simulink model "Demo5"  (Simulink 6.5)
settings: Solver=ode23t  SolverMode=SingleTasking  StartTime=0.0  StopTime=0.2  MaxStep=5e-5  RelTol=1e-3  AbsTol=1e-2
undefined symbols (not defined in the file): powergui
libraries: powerlib x5, powerlib_extras x2
settings Model: Creator=sybille  LastModifiedBy=PC_0  ExtModeTrigMode=oneshot  ExtModeArmWhenConnect=off  ExtModeAutoUpdateStatusClock=off  ProdHWDeviceType=Specified
settings DataIOCC: Decimation=10  LimitDataPoints=off  SaveFinalState=on  SaveOutput=off  SignalLoggingName=sigsOut
settings OptimizationCC: BlockReduction=off  BooleanDataType=off  InlineInvariantSignals=on
settings DebuggingCC: CheckExecutionContextPreStartOutputMsg=on  CheckExecutionContextRuntimeOutputMsg=on  SolverPrmCheckMsg=none  MultiTaskDSMMsg=warning  MultiTaskCondExecSysMsg=none  SigSpecEnsureSampleTimeMsg=none  UnconnectedInputMsg=none  UnconnectedOutputMsg=none  StrictBusMsg=None
settings HardwareCC: ProdHWDeviceType=Specified  TargetUnknown=on
settings RTWCC: IncludeERTFirstTime=on

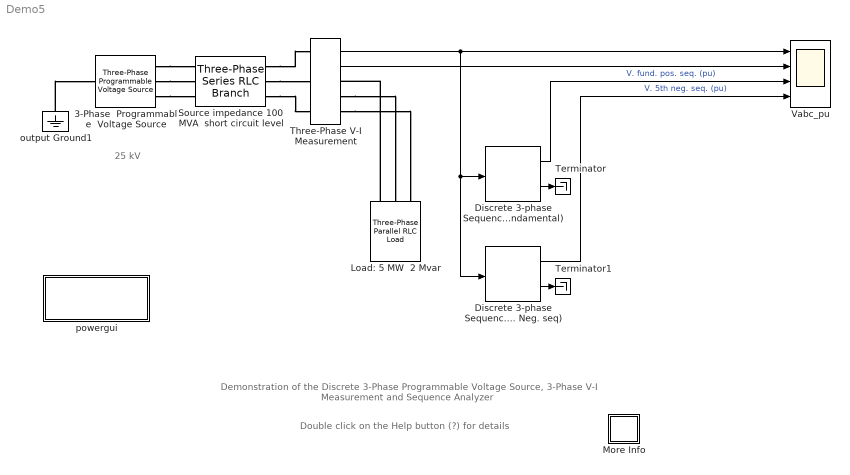
== system Demo5 ==
  note: Demonstration of the Discrete 3-Phase Programmable Voltage Source,
      |  3-Phase V-I Measurement and Sequence Analyzer
  note: Double click on the Help button (?) for details
  note: 25 kV
  3-Phase  Programmable  Voltage Source : powerlib/Electrical Sources/Three-Phase Programmable Voltage Source  DialogController=PMDialogs.PMDefaultMaskDlg  SystemSampleTime=-1  PositiveSequence="[25e3 0  60]"  VariationEntity=Amplitude  VariationType=Step  VariationStep=0.5  VariationRate=10  VariationMagnitude=0.3  VariationFrequency=2  VariationTiming=[0.05 1]  VariationPhaseA=off  Amplitudes=[1 0.8 1.2 1.0]  TimeValues=[0 0.1 0.15 0.2]  HarmonicGeneration=on  HarmonicA=[5 0.08 -45 2]  HarmonicB=[2 0 0 2]  Timing="[0.1  1]"
  Discrete 3-phase Sequence Analyzer (5th harm. Neg. seq) : powerlib_extras/Discrete Measurements/Discrete 3-phase Sequence Analyzer  DialogController=PMDialogs.PMDefaultMaskDlg  SystemSampleTime=-1  Freq=60  n=5  seq=Negative  Par_Init=[0 0]  Ts=50e-6
  Discrete 3-phase Sequence Analyzer (Fundamental) : powerlib_extras/Discrete Measurements/Discrete 3-phase Sequence Analyzer  DialogController=PMDialogs.PMDefaultMaskDlg  SystemSampleTime=-1  Freq=60  n=1  seq=Positive  Par_Init=[0 0]  Ts=50e-6
  Load: 5 MW  2 Mvar : powerlib/Elements/Three-Phase Parallel RLC Load  Orientation=down  DialogController=PMDialogs.PMDefaultMaskDlg  PhysicalDomain=powersysdomain  SubClassName=unknown  LeftPortType=p1  RightPortType=p1  LConnTagsString=A|B|C  Configuration=Y (grounded)  NominalVoltage=25e3  NominalFrequency=60  ActivePower=5e6  InductivePower=0  CapacitivePower=2e6  Measurements=None
  More Info : Subsystem
      settings: OpenFcn=showdemo(bdroot(gcb))
      mask Display: disp('?')
  Source impedance 100 MVA  short circuit level : powerlib/Elements/Three-Phase Series RLC Branch  DialogController=PMDialogs.PMDefaultMaskDlg  PhysicalDomain=powersysdomain  SubClassName=unknown  LeftPortType=p1  RightPortType=p1  LConnTagsString=A|B|C  RConnTagsString=A|B|C  BranchType=RL  Resistance=25^2/100/10  Inductance=25^2/100/377  Capacitance=[]  Measurements=None
  Terminator : Terminator
  Terminator1 : Terminator
  Three-Phase V-I Measurement : powerlib/Measurements/Three-Phase V-I Measurement  DialogController=PMDialogs.PMDefaultMaskDlg  SystemSampleTime=-1  VoltageMeasurement=phase-to-ground  SetLabelV=off  LabelV=V1  Vpu=on  CurrentMeasurement=yes  SetLabelI=off  LabelI=I1  Ipu=on  Pbase=10e6  Vbase=25e3  OutputType=Magnitude  PhasorSimulation=off  PSBequivalent=0
  Vabc_pu : Scope  NumInputPorts=4
      settings: TimeRange=0.2  YMin=-2~-2~0~0  YMax=2~1~2~0.2  DataFormat=Array  SampleInput=on
  output Ground1 : powerlib/Elements/Ground  Orientation=down  DialogController=PMDialogs.PMDefaultMaskDlg  PhysicalDomain=powersysdomain  SubClassName=unknown  LeftPortType=p1  RightPortType=p1  LConnTagsString=a
  powergui : Subsystem  Priority=2  AncestorBlock=powerlib/powergui  InitFcn=powergui( 'InitFcn_Callback' , gcb , 0 , [ ] );  mask(PSB option menu block){SimulationMode=Discrete, SampleTime=50e-6, echomessages=off, RestoreLinks=warning, x0status=blocks, Frange=[0:2:500], Ylog=off, Xlog=off, ShowGrid=off, save=off, variable=ZData, structure=, ZoomFFT=on, StartTime=0.0, cycles=1, DisplayStyle=off, fundamental=60, FreqAxis=off, MaxFrequency=1000, frequencyindice=60, frequencyindicesteady=1, RmsSteady=1, display=off, Ts=0, frequency=60, methode=off, HookPort=off, Interpol=off}
      mask prompts: SimulationMode "Simulation mode"; SampleTime "Sample time Ts (when simulation mode is Discrete) (s)"; echomessages "Echo  Messages"; RestoreLinks "Restore disabled links"; x0status "Initial electrical states status"; Frange "Impedance tool: Frequency Range"; Ylog "Impedance tool: Log impedance"; Xlog "Impedance tool: log Frequency"; ShowGrid "Impedance tool: grid"; save "Impedance tool: Save Data To Workspace"; variable "Impedance tool: Variable Name"; structure "Structure Name (PSBFFTSCOPE)"; ZoomFFT "ZoomFFT (PSBFFTSCOPE)"; StartTime "Start Time (PSBFFTSCOPE)"; cycles "Cycles (PSBFFTSCOPE)"; DisplayStyle "Display style (PSBFFTSCOPE)"; fundamental "Fundamental (PSBFFTSCOPE)"; FreqAxis "Frequency Axis (PSBFFTSCOPE)"; MaxFrequency "Max Frequency (PSBFFTSCOPE)"; frequencyindice "Load flow frequency (Hz)"; frequencyindicesteady "Frequency indice (STEADYSTATE)"; RmsSteady "RMS display (STEADYSTATE)"; display "Display Results"; Ts "OBSOLETE 1"; frequency "Phasor frequency (Hz)"; methode "Phasor simulation"; HookPort "Hook port"; Interpol "Interpolate"
      mask init:
      | powerlibroot = which('powersysdomain');
      | PSBroot = powerlibroot(1:end-16);
      | %
      | switch SimulationMode
      | 	case 1
      | 		message=sprintf('Continuous');
      | 	case 2
      |         SampleTimeeval=evalin('base',SampleTime,'NaN');
      |         if isnan(SampleTimeeval)
      |             message=sprintf('Warning !!,\nUndefined sample time');
      |         else
      |             message=sprintf('Discrete,\nTs = %.4g s.',SampleTimeeval);
      |         end
      | 	case 3
      | 		message=sprintf('Phasors');
      | end
      | if strcmp(bdroot,'powerlib')
      |   message='powergui';
      | end
      | power_initmask();
      settings: CopyFcn=powergui( 'Copy_Callback' , gcb , 0 , [ ] );  ModelCloseFcn=powergui( 'CloseButton_Callback' , gcb , [ ] , [ ] );  PreSaveFcn=powergui( 'CloseButton_Callback' , gcb , [ ] , [ ] );  NameChangeFcn=powergui( 'NameChangeFcn_Callback' , gcb , 0 , [ ] );
      settings: DeleteFcn=|
      | powergui( 'Copy_Callback' , gcb , 1 , [ ] );
      | powergui( 'CloseButton_Callback' , gcb , [ ] , [ ] );
      settings: OpenFcn=|
      | if (power_openblockproxy ('secondary'))
      | powergui(gcb,'PM')
      | end;
      mask Help: web(psbhelp)
      mask StyleString: popup(Continuous|Discrete|Phasor),edit,checkbox,popup(yes|warning|no),popup(blocks|steady|zero),edit,checkbox,checkbox,checkbox,checkbox,edit,edit,checkbox,edit,edit,edit,edit,checkbox,edit,edit,edit,edit,checkbox,edit,edit,checkbox,checkbox,checkbox
      mask CallbackString: ||||||||||||||||||||||||||powergui('HookPort',[],[],gcb);|
      mask Display: disp(message)
  wires:
  Discrete 3-phase Sequence Analyzer (Fundamental)/1 -> Vabc_pu/3  "V. fund. pos. seq. (pu)"
  Discrete 3-phase Sequence Analyzer (5th harm. Neg. seq)/1 -> Vabc_pu/4  "V. 5th neg. seq. (pu)"
  Discrete 3-phase Sequence Analyzer (Fundamental)/2 -> Terminator/1
  Discrete 3-phase Sequence Analyzer (5th harm. Neg. seq)/2 -> Terminator1/1
  Three-Phase V-I Measurement/2 -> Vabc_pu/2
  Three-Phase V-I Measurement/1 -> Vabc_pu/1, Discrete 3-phase Sequence Analyzer (Fundamental)/1, Discrete 3-phase Sequence Analyzer (5th harm. Neg. seq)/1
  connections:
  Source impedance 100 MVA  short circuit level/RConn1 -- Three-Phase V-I Measurement/LConn1
  Source impedance 100 MVA  short circuit level/RConn2 -- Three-Phase V-I Measurement/LConn2
  Source impedance 100 MVA  short circuit level/RConn3 -- Three-Phase V-I Measurement/LConn3
  3-Phase  Programmable  Voltage Source/RConn1 -- Source impedance 100 MVA  short circuit level/LConn1
  3-Phase  Programmable  Voltage Source/RConn2 -- Source impedance 100 MVA  short circuit level/LConn2
  3-Phase  Programmable  Voltage Source/RConn3 -- Source impedance 100 MVA  short circuit level/LConn3
  output Ground1/LConn1 -- 3-Phase  Programmable  Voltage Source/LConn1
  Load: 5 MW  2 Mvar/LConn1 -- Three-Phase V-I Measurement/RConn1
  Three-Phase V-I Measurement/RConn2 -- Load: 5 MW  2 Mvar/LConn2
  Three-Phase V-I Measurement/RConn3 -- Load: 5 MW  2 Mvar/LConn3

== system Demo5/More Info ==
  note: Circuit Description
  note: This demonstration ilustrates use of the 3-Phase Programmable Voltage Source,
      | 3-Phase V-I Measurement, and Sequence Analyzer blocks
  note: A  25kV, 100 MVA short-circuit level,  equivalent network feeds a 5MW, 2 Mvar capacitive load.
      |
      | The internal voltage of the source is controlled by the Discrete 3-phase Programmable Voltage Source block.
      |
      | Open the source dialog box and look at the parameters controlling the voltage. A positive-sequence of
      | 1.0 pu, 0 degrees is specified. At t = 0.05 s a step of 0.5 pu is applied on positive-sequence voltage magnitude,
      | then, at t = 0.1 s, 0.08 pu of 5th harmonic in negative sequence is added on the 1.5 pu voltage.
      |
      | In order to start simulation in steady state, the three voltage sources are initialized  with a
      | positive-sequence voltage of 25 kV, 0 degree, 60 Hz.
      |
      | The Three-Phase V-I Measurement block allows to monitor the three load voltages and currents.
      | Open its dialog box and see how this block allows to output the voltages and currents in pu.
      |
      | Two Discrete 3-phase Sequence Analyzer blocks are used to monitor the positive-sequeence of the three fundamental voltages Va, Vb, Vc
      | and the negative-sequence component of the 5th harmonic.
      |
      | The whole system, (power network, programmable source, and sequence analyzers) is discretized at a 50 us sample time.
  note: Demonstration
  note: Choose  Simulation/Start and observe the  voltage and current waveforms.
      |
      | The simulation starts in steady state with 1 pu voltage.
      | At t = 0.05 sec, the internal voltage is increased to 1.5 pu. At t = 0.10 sec. 0.08 pu of 5th harmonic internal voltage is added.
      |
      | Observe the fundamental component (pos. seq.) and the 5th harmonic component  (neg. seq.) measured by the two sequence analyzers.
      | The 0.08 pu 5th harmonic internal voltage is amplified at 0.14 pu at the load terminals.
      | As the sequence analyzers use Fourier analysis, their response time is one cycle.
  note: G. Sybille (Hydro-Quebec)

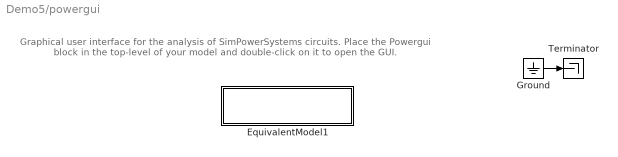
== system Demo5/powergui ==
  note: Graphical user interface for the analysis of  SimPowerSystems circuits.
      | Place the Powergui block in the top-level of your model and double-click
      | on it to open the GUI.
  EquivalentModel1 : Subsystem
      mask init:
      | SPS = get_param(gcbh,'UserData');
      | if isempty(SPS)
      | 	Ts=1;
      |     A=0;
      |     B=0;
      |     C=0;
      |     D=0;
      |     x0=0;
      | else
      | 	A=SPS.Adiscrete;
      |     B=SPS.Bdiscrete;
      |     C=SPS.Cdiscrete;
      |     D=SPS.Ddiscrete;
      |     x0=SPS.x0discrete;
      | 	Ts=SPS.PowerguiInfo.Ts;
      | end
      mask Display:
      | color('red')
      | disp('EQUIVALENT CIRCUIT')
  Ground : Ground
  Terminator : Terminator
  wires:
  Ground/1 -> Terminator/1

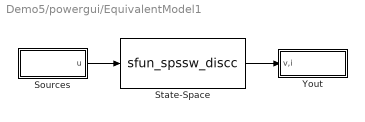
== system Demo5/powergui/EquivalentModel1 ==
  Sources : Subsystem
  State-Space : S-Function  FunctionName=sfun_spssw_discc  Parameters=Ts,A, B, C, D, x0
  Yout : Subsystem
  wires:
  Sources/1(u) -> State-Space/1
  State-Space/1 -> Yout/1(v,i)

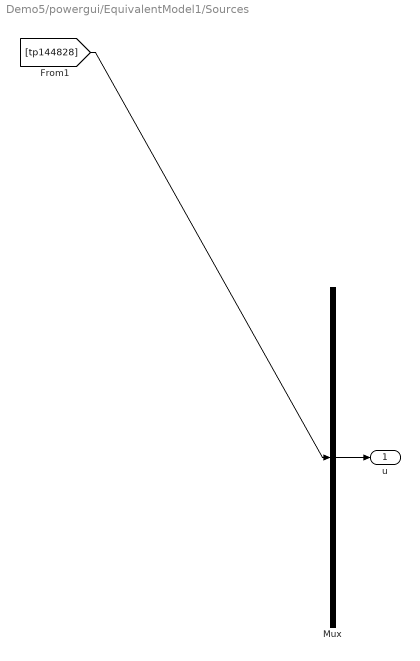
== system Demo5/powergui/EquivalentModel1/Sources ==
  Mux : Mux  Inputs=1
  u : Outport
  wires:
  Mux/1 -> u/1
  [tp144828] -> Mux/1

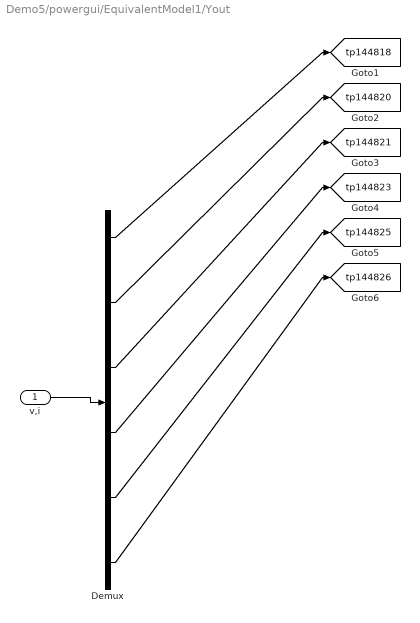
== system Demo5/powergui/EquivalentModel1/Yout ==
  v,i : Inport
  Demux : Demux  Outputs=[1 1 1 1 1 1]
  tag scope: tp144818=global, tp144820=global, tp144821=global, tp144823=global, tp144825=global, tp144826=global
  wires:
  v,i/1 -> Demux/1
  Demux/1 -> [tp144818]
  Demux/2 -> [tp144820]
  Demux/3 -> [tp144821]
  Demux/4 -> [tp144823]
  Demux/5 -> [tp144825]
  Demux/6 -> [tp144826]
